simulink library "tcan"  (Simulink 8.2)
settings: Solver=ode1  StartTime=0.0  StopTime=Inf  FixedStep=0.001  RelTol=1e-3
PostLoadFcn:
  | , if any(exist('dsrtsu_mdlpostloadfcn', 'file') == [2, 3, 6]), try dsrtsu_mdlpostloadfcn('Execute', bdroot); catch fprintf('Error in PostLoadFcn (dsrtsu_mdlpostloadfcn) for model "%s":\n %s\n', bdroot, lasterr); end, end,
undefined symbols (not defined in the file): ENUM_TARGETTYPE_BICYCLE, ENUM_TARGETTYPE_MOTORBIKE, ENUM_TARGETTYPE_PED, ENUM_TARGETTYPE_TRUCK, ENUM_TARGETTYPE_VEHICLE
libraries: simulink x2
settings Model: DSRTSU_INTERNAL_RTI_VER=440  DSRTSU_INTERNAL_RTI_TYPE=rti1401  RTICANMMDATA=struct('GeneralSetupData',struct('modelroot','D:\HAITEC\SVN\trunk\ADAS_Softwares\HTDragon\software\sw_development\arch\app\tcan','generalsettings',struct('filesettings',struct('destfolder',struct('Name','RTICANMM_FILES','Check',1),'buildfolder',struct('Name','.','Check',1),'AbsDestfolder',struct('Name','D:\HAITEC\SVN\trunk\ADAS_Softwares\HTDragon\software\sw_development\arch\app\tcan\RTICANMM_FILES'),'AbsBuildfolder',struct('Name','D:\HAITEC\SVN\trunk\ADAS_Softwares\HTDragon\software\sw_development\arch\app\tcan'))),'options',struct('addpaths',1,'rmpaths',1,'addtrcexclusion',logical(1),'cannavigator',struct('checkmonitoring',0),'show_usrtrc',0,'use_usrtrc',0),'advanced',struct('options',[1 1 1 1 1 1 1 1 1 1 1 1 1 1 1 1 1 1 1 1 1 1 1 1 1 1 1 1 1 1 1 1 1 1 1 1 1 1 1 1 1 1 1 1 1 1 1 1 1 1 1 1 1 1 1 1 1 1 1 1 1 1 1 1 1 1 1 1 1 1 1 1 1 1 1 1 1 1 1 1 1 1 1 1 1 1 1 1 1 1 1 1 1 1 1 1 1 1 1 1]),'MPSetup',{{}},'modelname','tcan','block','tcan'))  DSRTSU_INTERNAL_RTIFPGA=30  Creator=14014  LastModifiedBy=14014

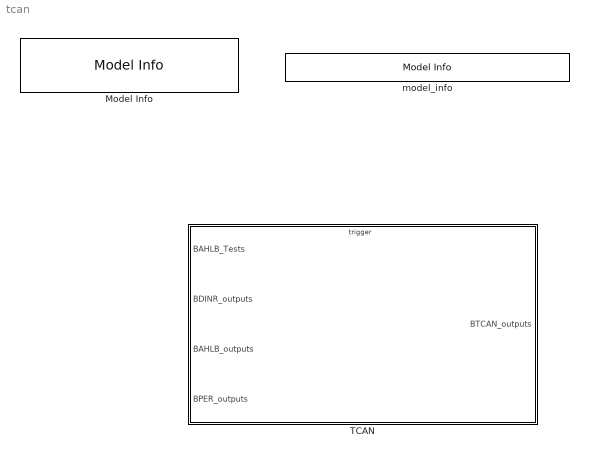
== system tcan ==
  Model Info : simulink/Model-Wide Utilities/Model Info  InitialBlockCM=None  BlockCM=None  Frame=on  DisplayStringWithTags=|  HorizontalTextAlignment=Left  LeftAlignmentValue=0.02  SourceBlockDiagram=tcan  TagMaxNumber=20
      | Model Version        : %<ModelVersion>
      | Creator                   : %<Creator>
      | Last Modified by    : %<LastModifiedBy>
  TCAN : Subsystem
  model_info : simulink/Model-Wide Utilities/Model Info  InitialBlockCM=None  BlockCM=None  Frame=on  DisplayStringWithTags=$Id: tcan.mdl 1497 2016-09-21 01:54:03Z bcluan $  HorizontalTextAlignment=Center  LeftAlignmentValue=0.5  SourceBlockDiagram=tcan  TagMaxNumber=20

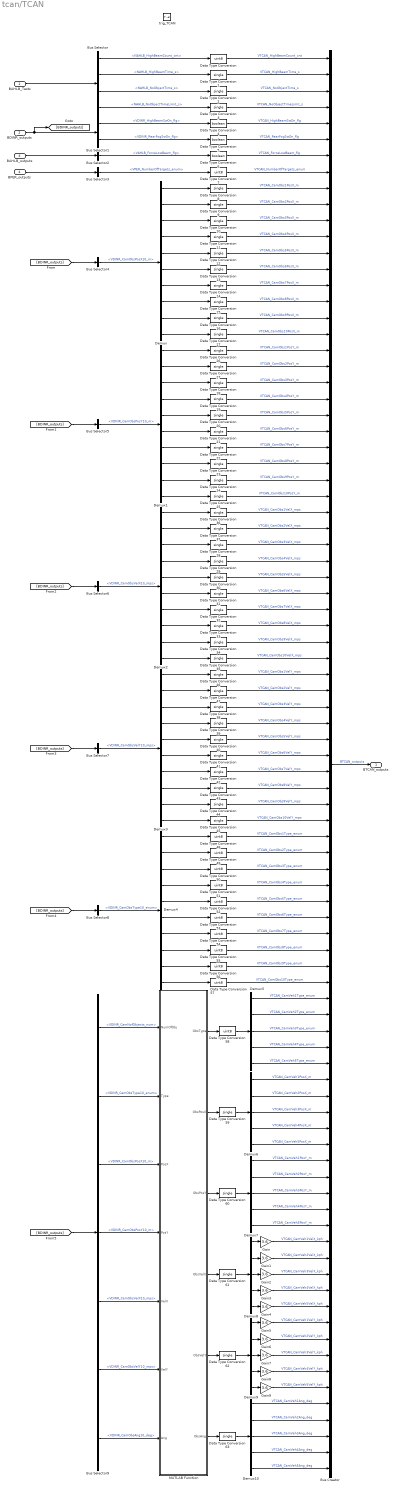
== system tcan/TCAN ==
  BAHLB_Tests : Inport
  BDINR_outputs : Inport  Port=2  OutDataTypeStr=Bus: BDINR_outputs
  BAHLB_outputs : Inport  Port=3  OutDataTypeStr=Bus: BAHLB_outputs
  BPER_outputs : Inport  Port=4  OutDataTypeStr=Bus: BPER_outputs
  trig_TCAN : TriggerPort  TriggerType=function-call
      settings: AttributesFormatString=State = %<StatesWhenEnabling>
  Bus Creator : BusCreator  Inputs=88
  Bus Selector : BusSelector  OutputSignals=NAHLB_HighBeamCount_cnt,NAHLB_HighBeamTime_s,NAHLB_NoObjectTime_s,NAHLB_NoObjectTimeLimit_s
  Bus Selector1 : BusSelector  OutputSignals=VDINR_HighBeamSwOn_flg,VDINR_RearFogSwOn_flg
  Bus Selector2 : BusSelector  OutputSignals=VAHLB_ForceLowBeam_flg
  Bus Selector3 : BusSelector  OutputSignals=VPER_NumberOfTargets_enum
  Bus Selector4 : BusSelector  OutputSignals=VDINR_CamObsPosX10_m
  Bus Selector5 : BusSelector  OutputSignals=VDINR_CamObsPosY10_m
  Bus Selector6 : BusSelector  OutputSignals=VDINR_CamObsVelX10_mps
  Bus Selector7 : BusSelector  OutputSignals=VDINR_CamObsVelY10_mps
  Bus Selector8 : BusSelector  OutputSignals=VDINR_CamObsType10_enum
  Bus Selector9 : BusSelector  OutputSignals=VDINR_CamNofObjects_num,VDINR_CamObsType10_enum,VDINR_CamObsPosX10_m,VDINR_CamObsPosY10_m,VDINR_CamObsVelX10_mps,VDINR_CamObsVelY10_mps,VDINR_CamObsAng10_deg
  Data Type Conversion{,7,48..58} (13 alike) : DataTypeConversion  OutDataTypeStr=uint8
  Data Type Conversion{1..3,8..47,59..63} (48 alike) : DataTypeConversion  OutDataTypeStr=single
  Data Type Conversion4 : DataTypeConversion  OutDataTypeStr=boolean
  Data Type Conversion5 : DataTypeConversion  OutDataTypeStr=boolean
  Data Type Conversion6 : DataTypeConversion  OutDataTypeStr=boolean
  Demux{,1..4} (5 alike) : Demux  Outputs=10
  Demux{5..10} (6 alike) : Demux  Outputs=5
  Gain{,1..9} (10 alike) : Gain  Gain=3.6
  MATLAB Function : MATLAB Function  TreatAsAtomicUnit=on
  BTCAN_outputs : Outport
  wires:
  Data Type Conversion55/1 -> Bus Creator/56  "VTCAN_CamObs8Type_enum"
  Data Type Conversion56/1 -> Bus Creator/57  "VTCAN_CamObs9Type_enum"
  Data Type Conversion49/1 -> Bus Creator/50  "VTCAN_CamObs2Type_enum"
  Data Type Conversion52/1 -> Bus Creator/53  "VTCAN_CamObs5Type_enum"
  Data Type Conversion57/1 -> Bus Creator/58  "VTCAN_CamObs10Type_enum"
  Data Type Conversion53/1 -> Bus Creator/54  "VTCAN_CamObs6Type_enum"
  Data Type Conversion54/1 -> Bus Creator/55  "VTCAN_CamObs7Type_enum"
  Data Type Conversion50/1 -> Bus Creator/51  "VTCAN_CamObs3Type_enum"
  Data Type Conversion51/1 -> Bus Creator/52  "VTCAN_CamObs4Type_enum"
  Data Type Conversion48/1 -> Bus Creator/49  "VTCAN_CamObs1Type_enum"
  Demux4/10 -> Data Type Conversion57/1
  Demux4/9 -> Data Type Conversion56/1
  Demux4/2 -> Data Type Conversion49/1
  Demux4/7 -> Data Type Conversion54/1
  Demux4/3 -> Data Type Conversion50/1
  Demux4/6 -> Data Type Conversion53/1
  Demux4/5 -> Data Type Conversion52/1
  Demux4/4 -> Data Type Conversion51/1
  Demux4/8 -> Data Type Conversion55/1
  Demux4/1 -> Data Type Conversion48/1
  Bus Selector8/1 -> Demux4/1  "<VDINR_CamObsType10_enum>"
  [BDINR_outputs] -> Bus Selector8/1
  Data Type Conversion39/1 -> Bus Creator/42  "VTCAN_CamObs4VelY_mps"
  Data Type Conversion43/1 -> Bus Creator/46  "VTCAN_CamObs8VelY_mps"
  Data Type Conversion41/1 -> Bus Creator/44  "VTCAN_CamObs6VelY_mps"
  Data Type Conversion42/1 -> Bus Creator/45  "VTCAN_CamObs7VelY_mps"
  Data Type Conversion40/1 -> Bus Creator/43  "VTCAN_CamObs5VelY_mps"
  Data Type Conversion47/1 -> Bus Creator/40  "VTCAN_CamObs2VelY_mps"
  Data Type Conversion44/1 -> Bus Creator/47  "VTCAN_CamObs9VelY_mps"
  Data Type Conversion45/1 -> Bus Creator/48  "VTCAN_CamObs10VelY_mps"
  Data Type Conversion46/1 -> Bus Creator/39  "VTCAN_CamObs1VelY_mps"
  Data Type Conversion38/1 -> Bus Creator/41  "VTCAN_CamObs3VelY_mps"
  Demux3/10 -> Data Type Conversion45/1
  Demux3/9 -> Data Type Conversion44/1
  Demux3/2 -> Data Type Conversion47/1
  Demux3/7 -> Data Type Conversion42/1
  Demux3/3 -> Data Type Conversion38/1
  Demux3/6 -> Data Type Conversion41/1
  Demux3/5 -> Data Type Conversion40/1
  Demux3/4 -> Data Type Conversion39/1
  Demux3/8 -> Data Type Conversion43/1
  Demux3/1 -> Data Type Conversion46/1
  Bus Selector7/1 -> Demux3/1  "<VDINR_CamObsVelY10_mps>"
  [BDINR_outputs] -> Bus Selector7/1
  Data Type Conversion30/1 -> Bus Creator/33  "VTCAN_CamObs5VelX_mps"
  Data Type Conversion33/1 -> Bus Creator/36  "VTCAN_CamObs8VelX_mps"
  Data Type Conversion36/1 -> Bus Creator/29  "VTCAN_CamObs1VelX_mps"
  Data Type Conversion32/1 -> Bus Creator/35  "VTCAN_CamObs7VelX_mps"
  Data Type Conversion31/1 -> Bus Creator/34  "VTCAN_CamObs6VelX_mps"
  Data Type Conversion34/1 -> Bus Creator/37  "VTCAN_CamObs9VelX_mps"
  Data Type Conversion35/1 -> Bus Creator/38  "VTCAN_CamObs10VelX_mps"
  Data Type Conversion37/1 -> Bus Creator/30  "VTCAN_CamObs2VelX_mps"
  Data Type Conversion28/1 -> Bus Creator/31  "VTCAN_CamObs3VelX_mps"
  Data Type Conversion29/1 -> Bus Creator/32  "VTCAN_CamObs4VelX_mps"
  Demux2/10 -> Data Type Conversion35/1
  Demux2/9 -> Data Type Conversion34/1
  Demux2/2 -> Data Type Conversion37/1
  Demux2/7 -> Data Type Conversion32/1
  Demux2/3 -> Data Type Conversion28/1
  Demux2/6 -> Data Type Conversion31/1
  Demux2/5 -> Data Type Conversion30/1
  Demux2/4 -> Data Type Conversion29/1
  Demux2/8 -> Data Type Conversion33/1
  Demux2/1 -> Data Type Conversion36/1
  Bus Selector6/1 -> Demux2/1  "<VDINR_CamObsVelX10_mps>"
  [BDINR_outputs] -> Bus Selector6/1
  Data Type Conversion26/1 -> Bus Creator/19  "VTCAN_CamObs1PosY_m"
  Data Type Conversion27/1 -> Bus Creator/20  "VTCAN_CamObs2PosY_m"
  Data Type Conversion25/1 -> Bus Creator/28  "VTCAN_CamObs10PosY_m"
  Data Type Conversion18/1 -> Bus Creator/21  "VTCAN_CamObs3PosY_m"
  Data Type Conversion22/1 -> Bus Creator/25  "VTCAN_CamObs7PosY_m"
  Data Type Conversion23/1 -> Bus Creator/26  "VTCAN_CamObs8PosY_m"
  Data Type Conversion21/1 -> Bus Creator/24  "VTCAN_CamObs6PosY_m"
  Data Type Conversion24/1 -> Bus Creator/27  "VTCAN_CamObs9PosY_m"
  Data Type Conversion19/1 -> Bus Creator/22  "VTCAN_CamObs4PosY_m"
  Data Type Conversion20/1 -> Bus Creator/23  "VTCAN_CamObs5PosY_m"
  Demux1/10 -> Data Type Conversion25/1
  Demux1/9 -> Data Type Conversion24/1
  Demux1/2 -> Data Type Conversion27/1
  Demux1/7 -> Data Type Conversion22/1
  Demux1/3 -> Data Type Conversion18/1
  Demux1/6 -> Data Type Conversion21/1
  Demux1/5 -> Data Type Conversion20/1
  Demux1/4 -> Data Type Conversion19/1
  Demux1/8 -> Data Type Conversion23/1
  Demux1/1 -> Data Type Conversion26/1
  Bus Selector5/1 -> Demux1/1  "<VDINR_CamObsPosY10_m>"
  Data Type Conversion17/1 -> Bus Creator/18  "VTCAN_CamObs10PosX_m"
  Data Type Conversion16/1 -> Bus Creator/17  "VTCAN_CamObs9PosX_m"
  Data Type Conversion15/1 -> Bus Creator/16  "VTCAN_CamObs8PosX_m"
  Data Type Conversion14/1 -> Bus Creator/15  "VTCAN_CamObs7PosX_m"
  Data Type Conversion13/1 -> Bus Creator/14  "VTCAN_CamObs6PosX_m"
  Data Type Conversion12/1 -> Bus Creator/13  "VTCAN_CamObs5PosX_m"
  Data Type Conversion11/1 -> Bus Creator/12  "VTCAN_CamObs4PosX_m"
  Data Type Conversion10/1 -> Bus Creator/11  "VTCAN_CamObs3PosX_m"
  Data Type Conversion9/1 -> Bus Creator/10  "VTCAN_CamObs2PosX_m"
  Data Type Conversion8/1 -> Bus Creator/9  "VTCAN_CamObs1PosX_m"
  Demux/10 -> Data Type Conversion17/1
  Demux/9 -> Data Type Conversion16/1
  Demux/2 -> Data Type Conversion9/1
  Demux/7 -> Data Type Conversion14/1
  Demux/3 -> Data Type Conversion10/1
  Demux/6 -> Data Type Conversion13/1
  Demux/5 -> Data Type Conversion12/1
  Demux/4 -> Data Type Conversion11/1
  Demux/8 -> Data Type Conversion15/1
  Demux/1 -> Data Type Conversion8/1
  Bus Selector4/1 -> Demux/1  "<VDINR_CamObsPosX10_m>"
  Data Type Conversion7/1 -> Bus Creator/8  "VTCAN_NumberOfTargets_enum"
  Bus Selector3/1 -> Data Type Conversion7/1  "<VPER_NumberOfTargets_enum>"
  Data Type Conversion6/1 -> Bus Creator/7  "VTCAN_ForceLowBeam_flg"
  Bus Selector2/1 -> Data Type Conversion6/1  "<VAHLB_ForceLowBeam_flg>"
  [BDINR_outputs] -> Bus Selector5/1
  [BDINR_outputs] -> Bus Selector4/1
  BPER_outputs/1 -> Bus Selector3/1
  BAHLB_outputs/1 -> Bus Selector2/1
  Data Type Conversion5/1 -> Bus Creator/6  "VTCAN_RearFogSwOn_flg"
  Data Type Conversion4/1 -> Bus Creator/5  "VTCAN_HighBeamSwOn_flg"
  Bus Selector1/2 -> Data Type Conversion5/1  "<VDINR_RearFogSwOn_flg>"
  Bus Selector1/1 -> Data Type Conversion4/1  "<VDINR_HighBeamSwOn_flg>"
  BDINR_outputs/1 -> Bus Selector1/1, [BDINR_outputs]
  Data Type Conversion3/1 -> Bus Creator/4  "VTCAN_NoObjectTimeLimit_s"
  Data Type Conversion2/1 -> Bus Creator/3  "VTCAN_NoObjectTime_s"
  Data Type Conversion1/1 -> Bus Creator/2  "VTCAN_HighBeamTime_s"
  Data Type Conversion/1 -> Bus Creator/1  "VTCAN_HighBeamCount_cnt"
  Bus Selector/4 -> Data Type Conversion3/1  "<NAHLB_NoObjectTimeLimit_s>"
  Bus Selector/3 -> Data Type Conversion2/1  "<NAHLB_NoObjectTime_s>"
  Bus Selector/2 -> Data Type Conversion1/1  "<NAHLB_HighBeamTime_s>"
  Bus Selector/1 -> Data Type Conversion/1  "<NAHLB_HighBeamCount_cnt>"
  BAHLB_Tests/1 -> Bus Selector/1
  Bus Creator/1 -> BTCAN_outputs/1  "BTCAN_outputs"
  [BDINR_outputs] -> Bus Selector9/1
  Bus Selector9/2 -> MATLAB Function/2(Type)  "<VDINR_CamObsType10_enum>"
  Bus Selector9/1 -> MATLAB Function/1(NumOfObj)  "<VDINR_CamNofObjects_num>"
  Bus Selector9/3 -> MATLAB Function/3(PosX)  "<VDINR_CamObsPosX10_m>"
  Bus Selector9/4 -> MATLAB Function/4(PosY)  "<VDINR_CamObsPosY10_m>"
  Bus Selector9/5 -> MATLAB Function/5(VelX)  "<VDINR_CamObsVelX10_mps>"
  Bus Selector9/6 -> MATLAB Function/6(VelY)  "<VDINR_CamObsVelY10_mps>"
  Bus Selector9/7 -> MATLAB Function/7(Ang)  "<VDINR_CamObsAng10_deg>"
  MATLAB Function/1(ObsType) -> Data Type Conversion58/1
  Data Type Conversion58/1 -> Demux5/1
  Demux5/4 -> Bus Creator/62  "VTCAN_CamVeh4Type_enum"
  Demux5/5 -> Bus Creator/63  "VTCAN_CamVeh5Type_enum"
  Demux5/1 -> Bus Creator/59  "VTCAN_CamVeh1Type_enum"
  Demux5/3 -> Bus Creator/61  "VTCAN_CamVeh3Type_enum"
  Demux5/2 -> Bus Creator/60  "VTCAN_CamVeh2Type_enum"
  Demux6/5 -> Bus Creator/68  "VTCAN_CamVeh5PosX_m"
  Demux6/4 -> Bus Creator/67  "VTCAN_CamVeh4PosX_m"
  Demux6/3 -> Bus Creator/66  "VTCAN_CamVeh3PosX_m"
  Demux6/1 -> Bus Creator/64  "VTCAN_CamVeh1PosX_m"
  Demux6/2 -> Bus Creator/65  "VTCAN_CamVeh2PosX_m"
  MATLAB Function/2(ObsPosX) -> Data Type Conversion59/1
  Data Type Conversion59/1 -> Demux6/1
  Demux7/5 -> Bus Creator/73  "VTCAN_CamVeh5PosY_m"
  Demux7/4 -> Bus Creator/72  "VTCAN_CamVeh4PosY_m"
  Demux7/3 -> Bus Creator/71  "VTCAN_CamVeh3PosY_m"
  Demux7/1 -> Bus Creator/69  "VTCAN_CamVeh1PosY_m"
  Demux7/2 -> Bus Creator/70  "VTCAN_CamVeh2PosY_m"
  Data Type Conversion60/1 -> Demux7/1
  MATLAB Function/3(ObsPosY) -> Data Type Conversion60/1
  Gain4/1 -> Bus Creator/78  "VTCAN_CamVeh5VelX_kph"
  Gain3/1 -> Bus Creator/77  "VTCAN_CamVeh4VelX_kph"
  Gain2/1 -> Bus Creator/76  "VTCAN_CamVeh3VelX_kph"
  Gain/1 -> Bus Creator/74  "VTCAN_CamVeh1VelX_kph"
  Gain1/1 -> Bus Creator/75  "VTCAN_CamVeh2VelX_kph"
  MATLAB Function/4(ObsVelX) -> Data Type Conversion61/1
  Gain9/1 -> Bus Creator/83  "VTCAN_CamVeh5VelY_kph"
  Gain8/1 -> Bus Creator/82  "VTCAN_CamVeh4VelY_kph"
  Gain7/1 -> Bus Creator/81  "VTCAN_CamVeh3VelY_kph"
  Gain5/1 -> Bus Creator/79  "VTCAN_CamVeh1VelY_kph"
  Gain6/1 -> Bus Creator/80  "VTCAN_CamVeh2VelY_kph"
  MATLAB Function/5(ObsVelY) -> Data Type Conversion62/1
  Demux10/5 -> Bus Creator/88  "VTCAN_CamVeh5Ang_deg"
  Demux10/4 -> Bus Creator/87  "VTCAN_CamVeh4Ang_deg"
  Demux10/3 -> Bus Creator/86  "VTCAN_CamVeh3Ang_deg"
  Demux10/1 -> Bus Creator/84  "VTCAN_CamVeh1Ang_deg"
  Demux10/2 -> Bus Creator/85  "VTCAN_CamVeh2Ang_deg"
  Data Type Conversion63/1 -> Demux10/1
  MATLAB Function/6(ObsAng) -> Data Type Conversion63/1
  Demux8/1 -> Gain/1
  Demux8/2 -> Gain1/1
  Demux8/3 -> Gain2/1
  Demux8/4 -> Gain3/1
  Demux8/5 -> Gain4/1
  Data Type Conversion61/1 -> Demux8/1
  Data Type Conversion62/1 -> Demux9/1
  Demux9/2 -> Gain6/1
  Demux9/5 -> Gain9/1
  Demux9/1 -> Gain5/1
  Demux9/3 -> Gain7/1
  Demux9/4 -> Gain8/1

== matlab function TCAN/MATLAB Function ==
  data: NumOfObj input double; ObsType output uint8 size=5; Type input double; PosX input double; PosY input double; VelX input double; VelY input double; Ang input double; ObsPosX output single size=5; ObsPosY output single size=5; ObsVelX output single size=5; ObsVelY output single size=5; ObsAng output single size=5; ENUM_TARGETTYPE_VEHICLE parameter double; ENUM_TARGETTYPE_TRUCK parameter double; ENUM_TARGETTYPE_MOTORBIKE parameter double; ENUM_TARGETTYPE_BICYCLE parameter double; ENUM_TARGETTYPE_PED parameter double
function [ObsType,ObsPosX, ObsPosY, ObsVelX, ObsVelY, ObsAng] = fcn(NumOfObj, Type, PosX, PosY, VelX, VelY, Ang, ENUM_TARGETTYPE_VEHICLE, ENUM_TARGETTYPE_TRUCK, ENUM_TARGETTYPE_MOTORBIKE, ENUM_TARGETTYPE_BICYCLE, ENUM_TARGETTYPE_PED)

j=1;
Typeall=uint8(7.*ones(5,1));
PosXall=single(0).*ones(5,1);
PosYall=single(0).*ones(5,1);
VelXall=single(0).*ones(5,1);
VelYall=single(0).*ones(5,1);
Angall=single(0).*ones(5,1);
for i=1:NumOfObj
    if (Type(i)==ENUM_TARGETTYPE_VEHICLE || ENUM_TARGETTYPE_TRUCK) && PosX(i)~=0
        Typeall(j)=Type(i);
        PosXall(j)=PosX(i);
        PosYall(j)=PosY(i);
        VelXall(j)=VelX(i);
        VelYall(j)=VelY(i);
        Angall(j)=Ang(i);
        j=j+1;
    end
    if j>=6
        break;
    end
end
if j<6
    for i=1:NumOfObj
        if (Type(i)==ENUM_TARGETTYPE_MOTORBIKE) && PosX(i)~=0
            Typeall(j)=Type(i);
            PosXall(j)=PosX(i);
            PosYall(j)=PosY(i);
            VelXall(j)=VelX(i);
            VelYall(j)=VelY(i);
            Angall(j)=Ang(i);
            j=j+1;
        end
        if j>=6
            break;
        end       
    end
end
if j<6
    for i=1:NumOfObj
        if (Type(i)==ENUM_TARGETTYPE_BICYCLE) && PosX(i)~=0
            Typeall(j)=Type(i);
            PosXall(j)=PosX(i);
            PosYall(j)=PosY(i);
            VelXall(j)=VelX(i);
            VelYall(j)=VelY(i);
            Angall(j)=Ang(i);
            j=j+1;
        end
        if j>=6
            break;
        end       
    end
end
if j<6
    for i=1:NumOfObj
        if (Type(i)==ENUM_TARGETTYPE_PED) && PosX(i)~=0
            Typeall(j)=Type(i);
            PosXall(j)=PosX(i);
            PosYall(j)=PosY(i);
            VelXall(j)=VelX(i);
            VelYall(j)=VelY(i);
            Angall(j)=Ang(i);
            j=j+1;
        end
        if j>=6
            break;
        end       
    end
end

ObsType = Typeall;
ObsPosX = PosXall;
ObsPosY = PosYall;
ObsVelX = VelXall;
ObsVelY = VelYall;
ObsAng = Angall;
